simulink model "s_cd_hmc_v2_pol0"  (R2016b)
(part 2 of 34)

  Counter3/1 -> pipeline28/1(d)
  pipeline28/1(q) -> valid80_cnt/1(out_reg)
  pipeline44/1(q) -> valid80/1(out_reg)
  Register2/1 -> pipeline44/1(d)
  pipeline100/1(q) -> Counter3/1
  pipeline80/1(q) -> Counter3/2
  [sys_rst] -> edge_detect6/1
  [valid80_local] -> edge_detect5/1
  edge_detect5/1 -> pipeline90/1(d), pipeline80/1(d)
  edge_detect6/1 -> pipeline100/1(d), pipeline47/1(d)
  edge_detect9/1 -> pipeline101/1(d), pipeline115/1(d)
  edge_detect11/1 -> pipeline20/1(d), pipeline116/1(d)
  pipeline17/1(q) -> [man_sync]
  Delay/1 -> man_sync/1(sim_1)
  Delay10/1 -> dvalid/1(sim_1)
  bus_expand1/8(lsb_out1) -> pipeline176/1(d)  "hmc_out16"
  pipeline222/1(q) -> bus_expand1/1(bus_in)
  [cd_in] -> pipeline222/1(d)
  pipeline176/1(q) -> cd_in/8(in_d07)
  pipeline175/1(q) -> cd_in/7(in_d06)
  pipeline172/1(q) -> cd_in/6(in_d05)
  pipeline171/1(q) -> cd_in/5(in_d04)
  pipeline170/1(q) -> cd_in/4(in_d03)
  pipeline169/1(q) -> cd_in/3(in_d02)
  pipeline168/1(q) -> cd_in/2(in_d01)
  bus_expand1/7(out2) -> pipeline175/1(d)
  bus_expand1/5(out4) -> pipeline171/1(d)
  bus_expand1/4(out5) -> pipeline170/1(d)
  bus_expand1/6(out3) -> pipeline172/1(d)
  bus_expand1/3(out6) -> pipeline169/1(d)
  bus_expand1/2(out7) -> pipeline168/1(d)
  pipeline19/1(q) -> pipeline178/1(d), Logical/1
  pipeline178/1(q) -> cd_in/9(in_dvalid)
  pipeline177/1(q) -> cd_in/10(in_sync)
  bus_expand1/1(msb_out8) -> pipeline87/1(d)
  pipeline87/1(q) -> cd_in/1(in_d00)
  [valid80_cd] -> pipeline19/1(d)
  [sync80_cd] -> pipeline15/1(d)
  pipeline15/1(q) -> pipeline177/1(d), pipeline57/1(d), Logical/2
  pipeline57/1(q) -> cd_in/12(trig)
  pipeline18/1(q) -> cd_in/11(we)
  Logical/1 -> pipeline18/1(d)
  pipeline81/1(q) -> cd_out/12(trig)
  pipeline78/1(q) -> cd_out/11(we)
  Logical1/1 -> pipeline78/1(d)
  pipeline79/1(q) -> pipeline81/1(d), Logical1/2, pipeline74/1(d)
  pipeline77/1(q) -> pipeline75/1(d), Logical1/1
  Counter5/1 -> Gateway Out27/1, Relational1/1
  Constant32/1 -> Relational1/2
  Gateway Out15/1 -> To Workspace42/1
  Gateway Out1/1 -> To Workspace1/1
  Delay1/1 -> Delay3/1
  Delay7/1 -> Delay12/1
  Gateway Out4/1 -> To Workspace10/1
  Delay9/1 -> Delay13/1
  [valid80] -> Terminator1/1
  Mux1/1 -> edge_detect12/1
  Delay3/1 -> Gateway Out28/1, Mux2/2
  [sync_select] -> Mux2/1, Gateway Out25/1, Mux1/1
  [dvalid] -> Logical16/3
  Register3/1 -> Delay8/1, Gateway Out29/1, Inverter3/1
  Delay6/1 -> Delay17/1
  Delay8/1 -> Delay1/1
  Gateway Out24/1 -> To Workspace35/1
  Gateway Out25/1 -> To Workspace36/1
  Gateway Out26/1 -> To Workspace37/1
  Gateway Out27/1 -> To Workspace40/1
  Register4/1 -> Delay7/1, Delay5/1, Delay2/1, Logical2/1
  Mux2/1 -> Delay14/1
  Gateway Out28/1 -> To Workspace41/1
  Delay4/1 -> Mux2/3
  Relational1/1 -> Mux1/3, Gateway Out24/1
  Delay17/1 -> Gateway Out26/1, Mux1/2
  edge_detect/1 -> Delay9/1
  Counter6/1 -> Slice1/1, Gateway Out31/1
  Slice1/1 -> Register3/3, Register3/1, Gateway Out30/1, edge_detect/1
  Gateway Out29/1 -> To Workspace9/1
  Gateway Out30/1 -> To Workspace33/1
  Gateway Out31/1 -> To Workspace34/1
  [sys_rst] -> Counter5/1, Counter6/1, Register3/2, Gateway Out33/1, Register4/2
  Inverter3/1 -> Logical2/2
  Logical16/1 -> Register4/3, Delay11/1, Gateway Out32/1, Register4/1
  Gateway Out32/1 -> To Workspace43/1
  Gateway Out33/1 -> To Workspace44/1
  Logical2/1 -> Counter6/2
  Delay2/1 -> Counter5/2
  Delay5/1 -> Relational1/3
  edge_detect12/1 -> [sync80_local], Gateway Out1/1
  [man_sync] -> Mux1/4
  Delay11/1 -> Mux2/4
  [hmc_post] -> Logical16/1
  [hmc_init] -> Logical16/2
  Delay12/1 -> Gateway Out4/1, Delay4/1
  Delay13/1 -> Delay6/1
  pipeline66/1(q) -> pipeline30/1(d)
  pipeline8/1(q) -> pipeline9/1(d)
  Delay14/1 -> [valid80_local], Gateway Out15/1
  pipeline1/1(q) -> [addr_map_sel]
  Constant8/1 -> addr_map_sel/1(sim_1)
  addr_map_sel/1(in_reg) -> pipeline1/1(d)
  edge_detect7/1(out) -> pipeline3/1(d)
